simulink model "epidemia"  (R2019b)
settings: Solver=ode4  StartTime=0.0  StopTime=tk  FixedStep=1  RelTol=1e-3
values from neighbouring files (symbols this model uses):
  beta = 0.1    [glowny.m]
  N = 38e6    (= 38000000)    [glowny.m]    (also in glowny_wsp_var.m)
  Z0 = D0/eta    (= 70)    [glowny.m]    (also in glowny_wsp_var.m)
settings Model: Creator=marci  LastModifiedBy=marci

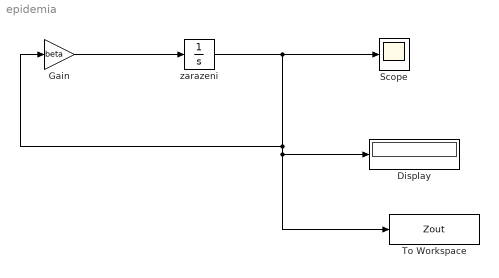
== system epidemia ==
  Display : Display
  Gain : Gain  Gain=beta
  Scope : Scope
  To Workspace : ToWorkspace  VariableName=Zout  SaveFormat=Timeseries  SampleTime=-1
  zarazeni : Integrator  InitialCondition=Z0  LimitOutput=on  UpperSaturationLimit=N  LowerSaturationLimit=0
  wires:
  Gain/1 -> zarazeni/1
  zarazeni/1 -> Display/1, To Workspace/1, Gain/1, Scope/1
